simulink model "simulacao"  (R2019a)
settings: Solver=VariableStepAuto  StartTime=0.0  StopTime=10.0  RelTol=1e-3
settings Model: Creator=Igorf  LastModifiedBy=Igorf

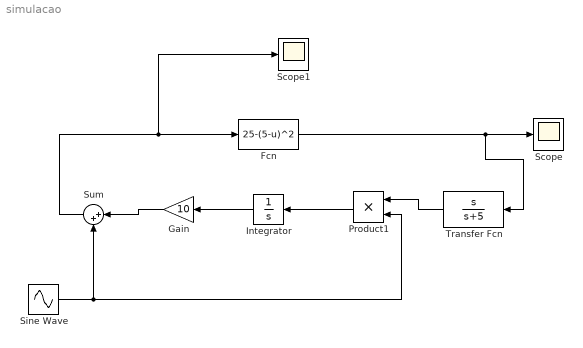
== system simulacao ==
  Fcn : Fcn  Expr=25-(5-u)^2
  Gain : Gain  Gain=10
  Integrator : Integrator
  Product1 : Product
  Scope : Scope
  Scope1 : Scope
  Sine Wave : Sin  Amplitude=0.2  Frequency=10*2*pi  SampleTime=0
  Sum : Sum  Inputs=|++
  Transfer Fcn : TransferFcn  Numerator=[1 0]  Denominator=[1 5]
  wires:
  Transfer Fcn/1 -> Product1/1
  Fcn/1 -> Scope/1, Transfer Fcn/1
  Sine Wave/1 -> Sum/2, Product1/2
  Product1/1 -> Integrator/1
  Integrator/1 -> Gain/1
  Gain/1 -> Sum/1
  Sum/1 -> Scope1/1, Fcn/1
